simulink model "observer2"  (R2019a)
settings: Solver=ode45  StartTime=0.0  StopTime=10.0  RelTol=1e-3
values from neighbouring files (symbols this model uses):
  A = [0, 1, 0, 0 ... (first row only)    [lab.m]
  B = [0 ... (first row only)    [lab.m]
  C = [1, 0, 0, 0 ... (first row only)    [lab.m]
  F = -acker(A, B, eign_F)    [lab.m]
  K = K2    [lab.m]
undefined symbols (not defined in the file or in its folder): A1
settings Model: Creator=ZIXUANXU  LastModifiedBy=ZIXUANXU
settings DataIOCC: ReturnWorkspaceOutputs=off  Refine=4

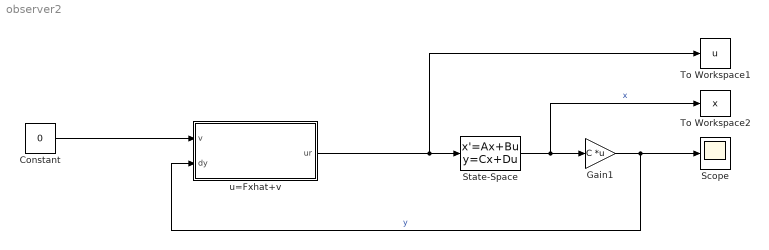
== system observer2 ==
  Constant : Constant  Value=0
  Gain1 : Gain  Gain=C  Multiplication=Matrix(K*u)
  Scope : Scope
  State-Space : StateSpace  A=A  B=B  C=eye(4)  D=zeros(4,1)  InitialCondition=[0.1 0 0.1 0]
  To Workspace1 : ToWorkspace  VariableName=u  SampleTime=-1
      settings: Save2DSignal=2-D array (concatenate along first dimension)
  To Workspace2 : ToWorkspace  VariableName=x  SampleTime=-1
      settings: Save2DSignal=2-D array (concatenate along first dimension)
  u=Fxhat+v : Subsystem
  wires:
  State-Space/1 -> To Workspace2/1, Gain1/1  "x"
  Gain1/1 -> u=Fxhat+v/2(dy), Scope/1  "y"
  u=Fxhat+v/1(ur) -> State-Space/1, To Workspace1/1
  Constant/1 -> u=Fxhat+v/1(v)

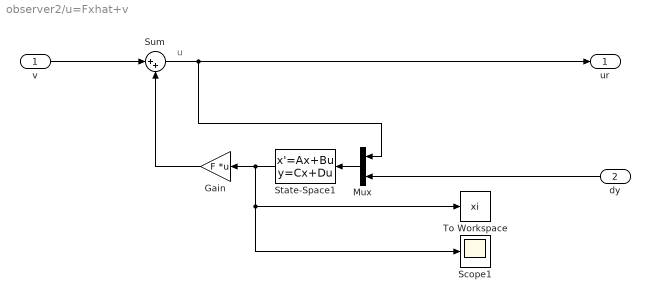
== system observer2/u=Fxhat+v ==
  note: u
  v : Inport
  dy : Inport  Port=2
  Gain : Gain  Gain=F  Multiplication=Matrix(K*u)
  Mux : Mux  Inputs=2
  Scope1 : Scope
  State-Space1 : StateSpace  A=A1  B=[B K]  C=eye(4)  D=zeros(4, 3)  InitialCondition=[0 0 0 0]
  Sum : Sum  Inputs=|++
  To Workspace : ToWorkspace  VariableName=xi  SampleTime=-1
      settings: Save2DSignal=2-D array (concatenate along first dimension)
  ur : Outport
  wires:
  v/1 -> Sum/1
  Sum/1 -> ur/1, Mux/1
  State-Space1/1 -> Scope1/1, To Workspace/1, Gain/1
  Gain/1 -> Sum/2
  Mux/1 -> State-Space1/1
  dy/1 -> Mux/2
